simulink model "SecRwLtStCalib"  (R2024b)
settings: Solver=FixedStepDiscrete  StartTime=0.0  StopTime=10.0  FixedStep=0.01  RelTol=1e-3
model workspace (MAT data in the model file):
  KeSMSwAcsMd6SecRwLtStBkReclnUpwdDnwdPos1Max_Val : Simulink.Parameter (value not decoded)
  KeSMSwAcsMd6SecRwLtStBkReclnUpwdDnwdPos1Min_Val : Simulink.Parameter (value not decoded)
  KeSMSwAcsMd6SecRwLtStBkReclnUpwdDnwdPos1_Val : Simulink.Parameter (value not decoded)
  KeSMSwAcsMd6SecRwLtStBkReclnUpwdDnwdPosMax_Val : Simulink.Parameter (value not decoded)
  KeSMSwAcsMd6SecRwLtStBkReclnUpwdDnwdPosMin_Val : Simulink.Parameter (value not decoded)
  KeSMSwAcsMd6SecRwLtStBkReclnUpwdDnwdPos_Val : Simulink.Parameter (value not decoded)
symbols that are objects in the model workspace (value not decoded): KeSMSwAcsMd6SecRwLtStBkReclnUpwdDnwdPos1_Val, KeSMSwAcsMd6SecRwLtStBkReclnUpwdDnwdPos1Max_Val, KeSMSwAcsMd6SecRwLtStBkReclnUpwdDnwdPos1Min_Val, KeSMSwAcsMd6SecRwLtStBkReclnUpwdDnwdPos_Val, KeSMSwAcsMd6SecRwLtStBkReclnUpwdDnwdPosMax_Val, KeSMSwAcsMd6SecRwLtStBkReclnUpwdDnwdPosMin_Val
undefined symbols (not defined in the file or in its folder): KeSMSw4SAcsMd21SecRwLtStBkReclnUpwdDnwdPos_Val, KeSMSw4SAcsMd21SecRwLtStBkReclnUpwdDnwdPosMax_Val, KeSMSw4SAcsMd21SecRwLtStBkReclnUpwdDnwdPosMin_Val, KeSMSw4SAcsMd21SecRwLtStFrwdBkwdPos_Val, KeSMSw4SAcsMd21SecRwLtStFrwdBkwdPosMax_Val, KeSMSw4SAcsMd21SecRwLtStFrwdBkwdPosMin_Val, KeSMSw4SAcsMd21SecRwLtStHdrstFrwdBkwdPos_Val, KeSMSw4SAcsMd21SecRwLtStHdrstFrwdBkwdPosMax_Val, KeSMSw4SAcsMd21SecRwLtStHdrstFrwdBkwdPosMin_Val, KeSMSw4SAcsMd21SecRwLtStHdrstUpwdDnwdPos_Val, KeSMSw4SAcsMd21SecRwLtStHdrstUpwdDnwdPosMax_Val, KeSMSw4SAcsMd21SecRwLtStHdrstUpwdDnwdPosMin_Val, KeSMSw4SAcsMd22SecRwLtStBkReclnUpwdDnwdPos1_Val, KeSMSw4SAcsMd22SecRwLtStBkReclnUpwdDnwdPos2_Val, KeSMSw4SAcsMd22SecRwLtStBkReclnUpwdDnwdPos2Max_Val, KeSMSw4SAcsMd22SecRwLtStBkReclnUpwdDnwdPos2Min_Val, KeSMSw4SAcsMd22SecRwLtStBkReclnUpwdDnwdPosMax_Val, KeSMSw4SAcsMd22SecRwLtStBkReclnUpwdDnwdPosMin_Val, KeSMSw4SAcsMd22SecRwLtStFrwdBkwdPos_Val, KeSMSw4SAcsMd22SecRwLtStFrwdBkwdPosMax_Val, KeSMSw4SAcsMd22SecRwLtStFrwdBkwdPosMin_Val, KeSMSw4SAcsMd22SecRwLtStFtrstUpwdDnwdPos_Val, KeSMSw4SAcsMd22SecRwLtStFtrstUpwdDnwdPosMax_Val, KeSMSw4SAcsMd22SecRwLtStFtrstUpwdDnwdPosMin_Val, KeSMSw4SAcsMd22SecRwLtStHdrstFrwdBkwdPos_Val, KeSMSw4SAcsMd22SecRwLtStHdrstFrwdBkwdPosMax_Val, KeSMSw4SAcsMd22SecRwLtStHdrstFrwdBkwdPosMin_Val, KeSMSw4SAcsMd22SecRwLtStHdrstUpwdDnwdPos_Val, KeSMSw4SAcsMd22SecRwLtStHdrstUpwdDnwdPosMax_Val, KeSMSw4SAcsMd22SecRwLtStHdrstUpwdDnwdPosMin_Val, KeSMSw4SAcsMd22SecRwLtStLegrstOtwdInwdPos_Val, KeSMSw4SAcsMd22SecRwLtStLegrstOtwdInwdPosMax_Val, KeSMSw4SAcsMd22SecRwLtStLegrstOtwdInwdPosMin_Val, KeSMSw4SAcsMd22SecRwLtStLegrstUpwdDnwdPos_Val, KeSMSw4SAcsMd22SecRwLtStLegrstUpwdDnwdPosMax_Val, KeSMSw4SAcsMd22SecRwLtStLegrstUpwdDnwdPosMin_Val, KeSMSw4SAcsMd25SecRwLtStBkReclnUpwdDnwdPos_Val, KeSMSw4SAcsMd25SecRwLtStBkReclnUpwdDnwdPosMax_Val, KeSMSw4SAcsMd25SecRwLtStBkReclnUpwdDnwdPosMin_Val, KeSMSw4SAcsMd25SecRwLtStFrwdBkwdPos_Val, KeSMSw4SAcsMd25SecRwLtStFrwdBkwdPosMax_Val, KeSMSw4SAcsMd25SecRwLtStFrwdBkwdPosMin_Val, KeSMSw4SAcsMd25SecRwLtStHdrstFrwdBkwdPos_Val, KeSMSw4SAcsMd25SecRwLtStHdrstFrwdBkwdPosMax_Val, KeSMSw4SAcsMd25SecRwLtStHdrstFrwdBkwdPosMin_Val, KeSMSw4SAcsMd25SecRwLtStHdrstUpwdDnwdPos_Val, KeSMSw4SAcsMd25SecRwLtStHdrstUpwdDnwdPosMax_Val, KeSMSw4SAcsMd25SecRwLtStHdrstUpwdDnwdPosMin_Val, KeSMSw4SAcsMd26SecRwLtStBkReclnUpwdDnwdPos_Val, KeSMSw4SAcsMd26SecRwLtStBkReclnUpwdDnwdPosMax_Val, KeSMSw4SAcsMd26SecRwLtStBkReclnUpwdDnwdPosMin_Val, KeSMSw4SAcsMd26SecRwLtStFrwdBkwdPos_Val, KeSMSw4SAcsMd26SecRwLtStFrwdBkwdPosMax_Val, KeSMSw4SAcsMd26SecRwLtStFrwdBkwdPosMin_Val, KeSMSw4SAcsMd26SecRwLtStFtrstUpwdDnwdPos_Val, KeSMSw4SAcsMd26SecRwLtStFtrstUpwdDnwdPosMax_Val, KeSMSw4SAcsMd26SecRwLtStFtrstUpwdDnwdPosMin_Val, KeSMSw4SAcsMd26SecRwLtStHdrstFrwdBkwdPos_Val, KeSMSw4SAcsMd26SecRwLtStHdrstFrwdBkwdPosMax_Val, KeSMSw4SAcsMd26SecRwLtStHdrstFrwdBkwdPosMin_Val ... (+496)
libraries: TrgtPosSelcLib x61, StIsPosChkLib x1, simulink x1
(part 8 of 8)

== system SecRwLtStCalib/SecRwLtStZeroTrgtPosSelc_1_Cal_sys/SecRwLtStZeroTrgtPosSelc_Cal_sys/Subsystem1 ==
  StNumFlg_Is6s_read : Inport
  Enable : EnablePort
  Constant : Constant  Value=4095  OutDataTypeStr=uint16
  Data Type Conversion : DataTypeConversion  SaturateOnIntegerOverflow=off  RndMeth=Floor
  Data Type Conversion1 : DataTypeConversion  SaturateOnIntegerOverflow=off  RndMeth=Floor
  Data Type Conversion2 : DataTypeConversion  SaturateOnIntegerOverflow=off  RndMeth=Floor
  PA_KeSMSw6SAcsEntrySecRwLtStCushnFrtUpwdDnwdPosMax_Val : Constant  Value=KeSMSw6SAcsEntrySecRwLtStCushnFrtUpwdDnwdPosMax_Val
  PA_KeSMSw6SAcsEntrySecRwLtStCushnFrtUpwdDnwdPosMin_Val : Constant  Value=KeSMSw6SAcsEntrySecRwLtStCushnFrtUpwdDnwdPosMin_Val
  PA_KeSMSw6SAcsEntrySecRwLtStCushnFrtUpwdDnwdPos_Val : Constant  Value=KeSMSw6SAcsEntrySecRwLtStCushnFrtUpwdDnwdPos_Val
  PA_KeSMSw6SAcsMd56SecRwLtStCushnFrtUpwdDnwdPosMax_Val : Constant  Value=KeSMSw6SAcsMd56SecRwLtStCushnFrtUpwdDnwdPosMax_Val
  PA_KeSMSw6SAcsMd56SecRwLtStCushnFrtUpwdDnwdPosMin_Val : Constant  Value=KeSMSw6SAcsMd56SecRwLtStCushnFrtUpwdDnwdPosMin_Val
  PA_KeSMSw6SAcsMd56SecRwLtStCushnFrtUpwdDnwdPos_Val : Constant  Value=KeSMSw6SAcsMd56SecRwLtStCushnFrtUpwdDnwdPos_Val
  PA_KeSMSw6SRecoveryMdSecRwLtStCushnFrtUpwdDnwdPosMax_Val : Constant  Value=KeSMSw6SRecoveryMdSecRwLtStCushnFrtUpwdDnwdPosMax_Val
  PA_KeSMSw6SRecoveryMdSecRwLtStCushnFrtUpwdDnwdPosMin_Val : Constant  Value=KeSMSw6SRecoveryMdSecRwLtStCushnFrtUpwdDnwdPosMin_Val
  PA_KeSMSw6SRecoveryMdSecRwLtStCushnFrtUpwdDnwdPos_Val : Constant  Value=KeSMSw6SRecoveryMdSecRwLtStCushnFrtUpwdDnwdPos_Val
  PA_KeSMSwAcsEntrySecRwLtStCushnFrtIUpwdDnwdPosMax_Val : Constant  Value=KeSMSwAcsEntrySecRwLtStCushnFrtIUpwdDnwdPosMax_Val
  PA_KeSMSwAcsEntrySecRwLtStCushnFrtIUpwdDnwdPosMin_Val : Constant  Value=KeSMSwAcsEntrySecRwLtStCushnFrtIUpwdDnwdPosMin_Val
  PA_KeSMSwAcsEntrySecRwLtStCushnFrtIUpwdDnwdPos_Val : Constant  Value=KeSMSwAcsEntrySecRwLtStCushnFrtIUpwdDnwdPos_Val
  PA_KeSMSwAcsMd56SecRwLtStCushnFrtUpwdDnwdPosMax_Val : Constant  Value=KeSMSwAcsMd56SecRwLtStCushnFrtUpwdDnwdPosMax_Val
  PA_KeSMSwAcsMd56SecRwLtStCushnFrtUpwdDnwdPosMin_Val : Constant  Value=KeSMSwAcsMd56SecRwLtStCushnFrtUpwdDnwdPosMin_Val
  PA_KeSMSwAcsMd56SecRwLtStCushnFrtUpwdDnwdPos_Val : Constant  Value=KeSMSwAcsMd56SecRwLtStCushnFrtUpwdDnwdPos_Val
  PA_KeSMSwAcsMd8SecRwLtStCushnFrtUpwdDnwdPosMax_Val : Constant  Value=KeSMSwAcsMd8SecRwLtStCushnFrtUpwdDnwdPosMax_Val
  PA_KeSMSwAcsMd8SecRwLtStCushnFrtUpwdDnwdPosMin_Val : Constant  Value=KeSMSwAcsMd8SecRwLtStCushnFrtUpwdDnwdPosMin_Val
  PA_KeSMSwAcsMd8SecRwLtStCushnFrtUpwdDnwdPos_Val : Constant  Value=KeSMSwAcsMd8SecRwLtStCushnFrtUpwdDnwdPos_Val
  PA_KeSMSwRecoveryMdSecRwLtStCushnFrtUpwdDnwdPosMax_Val : Constant  Value=KeSMSwRecoveryMdSecRwLtStCushnFrtUpwdDnwdPosMax_Val
  PA_KeSMSwRecoveryMdSecRwLtStCushnFrtUpwdDnwdPosMin_Val : Constant  Value=KeSMSwRecoveryMdSecRwLtStCushnFrtUpwdDnwdPosMin_Val
  PA_KeSMSwRecoveryMdSecRwLtStCushnFrtUpwdDnwdPos_Val : Constant  Value=KeSMSwRecoveryMdSecRwLtStCushnFrtUpwdDnwdPos_Val
  TrgtPosSelcNot4sMotor{,1..3} (4 alike) : TrgtPosSelcLib/TrgtPosSelcNo4sMd  SystemSampleTime=-1  VariantActivationTime=update diagram  AllowFlexibleInterface=on  Latency=0  AutoFrameSizeCalculation=off
  ComfortMdR2LZeroTrgtPosCalib_TrgtPosArray_write : Outport  VectorParamsAs1DForOutWhenUnconnected=off
      settings: EnsureOutportIsVirtual=on
  EZEMdR2LZeroTrgtPosCalib_TrgtPosArray_write : Outport  Port=2  VectorParamsAs1DForOutWhenUnconnected=off
      settings: EnsureOutportIsVirtual=on
  Md8R2LZeroTrgtPosCalib_TrgtPosArray_write : Outport  Port=3  VectorParamsAs1DForOutWhenUnconnected=off
      settings: EnsureOutportIsVirtual=on
  Md56R2LZeroTrgtPosCalib_TrgtPosArray_write : Outport  Port=4  VectorParamsAs1DForOutWhenUnconnected=off
      settings: EnsureOutportIsVirtual=on
  wires:
  [Is6s] -> TrgtPosSelcNot4sMotor2/1
  PA_KeSMSwAcsMd8SecRwLtStCushnFrtUpwdDnwdPos_Val/1 -> TrgtPosSelcNot4sMotor2/5
  PA_KeSMSwRecoveryMdSecRwLtStCushnFrtUpwdDnwdPos_Val/1 -> TrgtPosSelcNot4sMotor/5
  [invalidPos] -> TrgtPosSelcNot4sMotor2/3
  PA_KeSMSw6SAcsEntrySecRwLtStCushnFrtUpwdDnwdPosMax_Val/1 -> TrgtPosSelcNot4sMotor1/3
  PA_KeSMSwAcsEntrySecRwLtStCushnFrtIUpwdDnwdPosMin_Val/1 -> TrgtPosSelcNot4sMotor1/7
  Data Type Conversion2/1 -> Md56R2LZeroTrgtPosCalib_TrgtPosArray_write/1
  Data Type Conversion/1 -> ComfortMdR2LZeroTrgtPosCalib_TrgtPosArray_write/1
  PA_KeSMSwAcsEntrySecRwLtStCushnFrtIUpwdDnwdPosMax_Val/1 -> TrgtPosSelcNot4sMotor1/6
  PA_KeSMSwAcsEntrySecRwLtStCushnFrtIUpwdDnwdPos_Val/1 -> TrgtPosSelcNot4sMotor1/5
  PA_KeSMSw6SAcsEntrySecRwLtStCushnFrtUpwdDnwdPosMin_Val/1 -> TrgtPosSelcNot4sMotor1/4
  PA_KeSMSw6SAcsMd56SecRwLtStCushnFrtUpwdDnwdPos_Val/1 -> TrgtPosSelcNot4sMotor3/2
  TrgtPosSelcNot4sMotor2/1 -> Md8R2LZeroTrgtPosCalib_TrgtPosArray_write/1
  PA_KeSMSw6SAcsEntrySecRwLtStCushnFrtUpwdDnwdPos_Val/1 -> TrgtPosSelcNot4sMotor1/2
  [invalidPos] -> TrgtPosSelcNot4sMotor2/4
  [invalidPos] -> TrgtPosSelcNot4sMotor2/2
  PA_KeSMSwAcsMd8SecRwLtStCushnFrtUpwdDnwdPosMax_Val/1 -> TrgtPosSelcNot4sMotor2/6
  PA_KeSMSwRecoveryMdSecRwLtStCushnFrtUpwdDnwdPosMin_Val/1 -> TrgtPosSelcNot4sMotor/7
  PA_KeSMSwAcsMd8SecRwLtStCushnFrtUpwdDnwdPosMin_Val/1 -> TrgtPosSelcNot4sMotor2/7
  PA_KeSMSwAcsMd56SecRwLtStCushnFrtUpwdDnwdPosMin_Val/1 -> TrgtPosSelcNot4sMotor3/7
  StNumFlg_Is6s_read/1 -> [Is6s], TrgtPosSelcNot4sMotor1/1, TrgtPosSelcNot4sMotor/1
  TrgtPosSelcNot4sMotor1/1 -> Data Type Conversion1/1
  PA_KeSMSw6SRecoveryMdSecRwLtStCushnFrtUpwdDnwdPosMax_Val/1 -> TrgtPosSelcNot4sMotor/3
  TrgtPosSelcNot4sMotor/1 -> Data Type Conversion/1
  Data Type Conversion1/1 -> EZEMdR2LZeroTrgtPosCalib_TrgtPosArray_write/1
  PA_KeSMSwRecoveryMdSecRwLtStCushnFrtUpwdDnwdPosMax_Val/1 -> TrgtPosSelcNot4sMotor/6
  PA_KeSMSw6SRecoveryMdSecRwLtStCushnFrtUpwdDnwdPos_Val/1 -> TrgtPosSelcNot4sMotor/2
  PA_KeSMSw6SRecoveryMdSecRwLtStCushnFrtUpwdDnwdPosMin_Val/1 -> TrgtPosSelcNot4sMotor/4
  [Is6s] -> TrgtPosSelcNot4sMotor3/1
  PA_KeSMSwAcsMd56SecRwLtStCushnFrtUpwdDnwdPosMax_Val/1 -> TrgtPosSelcNot4sMotor3/6
  PA_KeSMSw6SAcsMd56SecRwLtStCushnFrtUpwdDnwdPosMax_Val/1 -> TrgtPosSelcNot4sMotor3/3
  PA_KeSMSwAcsMd56SecRwLtStCushnFrtUpwdDnwdPos_Val/1 -> TrgtPosSelcNot4sMotor3/5
  TrgtPosSelcNot4sMotor3/1 -> Data Type Conversion2/1
  PA_KeSMSw6SAcsMd56SecRwLtStCushnFrtUpwdDnwdPosMin_Val/1 -> TrgtPosSelcNot4sMotor3/4
  Constant/1 -> [invalidPos]
